simulink library "BaselineVehicleController_cl"  (R2020a)
settings: Solver=VariableStepAuto  StartTime=0.0  StopTime=10.0  RelTol=1e-3
undefined symbols (not defined in the file): best_gear, Clutch, dem_wheel_speed, dem_wheel_torque, Gear, ICE, MTC, Neg_RPM, Neg_T_eng_Nm, t_acc, tau_acc, TRAN, VEH
libraries: BaselineVelocityController_UL x1, Traffic_2_UL x1
settings Model: Creator=John Jr  LastModifiedBy=John Jr

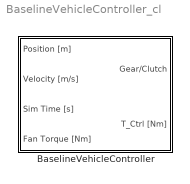
== system BaselineVehicleController_cl ==
  BaselineVehicleController : Subsystem

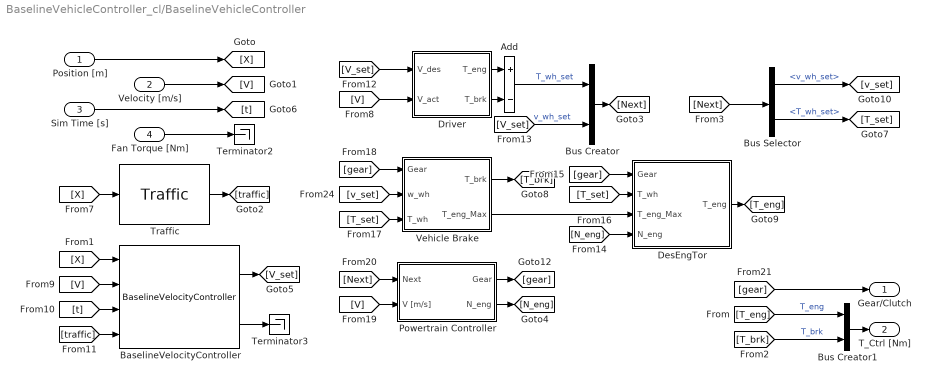
== system BaselineVehicleController_cl/BaselineVehicleController ==
  Position [m] : Inport
  Velocity [m/s] : Inport  Port=2
  Sim Time [s] : Inport  Port=3
  Fan Torque [Nm] : Inport  Port=4
  Add : Sum  Inputs=+-
  BaselineVelocityController : BaselineVelocityController_UL/BaselineVelocityController  SystemSampleTime=-1  Latency=0  AutoFrameSizeCalculation=off
  Bus Creator : BusCreator  Inputs=2
  Bus Creator1 : BusCreator  Inputs=2
  Bus Selector : BusSelector  OutputSignals=v_wh_set,T_wh_set
  DesEngTor : Subsystem
  Driver : Subsystem
  Powertrain Controller : Subsystem
  Terminator2 : Terminator
  Terminator3 : Terminator
  Traffic : Traffic_2_UL/Traffic  SystemSampleTime=-1  Latency=0  AutoFrameSizeCalculation=off
  Vehicle Brake : Subsystem
  Gear/Clutch : Outport  VectorParamsAs1DForOutWhenUnconnected=off
  T_Ctrl [Nm] : Outport  Port=2  VectorParamsAs1DForOutWhenUnconnected=off
  wires:
  Velocity [m/s]/1 -> [V]
  Position [m]/1 -> [X]
  Bus Selector/2 -> [T_set]  "<T_wh_set>"
  [Next] -> Bus Selector/1
  Bus Selector/1 -> [v_set]  "<v_wh_set>"
  Fan Torque [Nm]/1 -> Terminator2/1
  [gear] -> Gear/Clutch/1
  Bus Creator1/1 -> T_Ctrl [Nm]/1
  [X] -> Traffic/1
  Traffic/1 -> [traffic]
  Sim Time [s]/1 -> [t]
  [X] -> BaselineVelocityController/1
  [V] -> BaselineVelocityController/2
  [t] -> BaselineVelocityController/3
  [traffic] -> BaselineVelocityController/4
  Bus Creator/1 -> [Next]
  [V_set] -> Driver/1(V_des)
  [V_set] -> Bus Creator/2  "v_wh_set"
  Add/1 -> Bus Creator/1  "T_wh_set"
  Driver/2(T_brk) -> Add/2
  Driver/1(T_eng) -> Add/1
  [V] -> Driver/2(V_act)
  BaselineVelocityController/1 -> [V_set]
  BaselineVelocityController/2 -> Terminator3/1
  [gear] -> Vehicle Brake/1(Gear)
  [gear] -> DesEngTor/1(Gear)
  [v_set] -> Vehicle Brake/2(w_wh)
  Vehicle Brake/1(T_brk) -> [T_brk]
  [N_eng] -> DesEngTor/4(N_eng)
  [T_set] -> DesEngTor/2(T_wh)
  [T_set] -> Vehicle Brake/3(T_wh)
  Vehicle Brake/2(T_eng_Max) -> DesEngTor/3(T_eng_Max)
  DesEngTor/1(T_eng) -> [T_eng]
  [Next] -> Powertrain Controller/1(Next)
  Powertrain Controller/1(Gear) -> [gear]
  [V] -> Powertrain Controller/2(V [m/s])
  [T_eng] -> Bus Creator1/1  "T_eng"
  [T_brk] -> Bus Creator1/2  "T_brk"
  Powertrain Controller/2(N_eng) -> [N_eng]

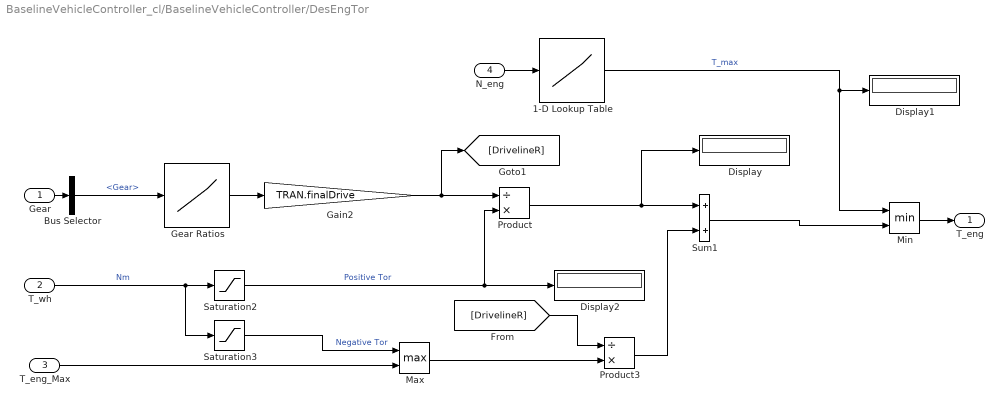
== system BaselineVehicleController_cl/BaselineVehicleController/DesEngTor ==
  Gear : Inport
  T_wh : Inport  Port=2
  T_eng_Max : Inport  Port=3
  N_eng : Inport  Port=4
  1-D Lookup Table : Lookup_n-D  NumberOfTableDimensions=1  BreakpointsForDimension1=MTC.espd  Table=MTC.T_max  InternalRulePriority=Speed  RndMeth=Simplest  InputSameDT=on
  Bus Selector : BusSelector  OutputSignals=Gear
  Display : Display
  Display1 : Display
  Display2 : Display
  Gain2 : Gain  Gain=TRAN.finalDrive
  Gear Ratios : Lookup_n-D  NumberOfTableDimensions=1  BreakpointsForDimension1=[1:TRAN.numGears]  Table=TRAN.gears  ExtrapMethod=Clip  UseLastTableValue=on  InternalRulePriority=Speed  RndMeth=Simplest  InputSameDT=on
  Max : MinMax  Function=max  Inputs=2
  Min : MinMax  Inputs=2
  Product : Product  Inputs=/*
  Product3 : Product  Inputs=/*
  Saturation2 : Saturate  UpperLimit=inf  LowerLimit=0
  Saturation3 : Saturate  UpperLimit=0  LowerLimit=-inf
  Sum1 : Sum
  T_eng : Outport  VectorParamsAs1DForOutWhenUnconnected=off
  wires:
  Gain2/1 -> [DrivelineR], Product/1
  Product/1 -> Display/1, Sum1/1
  T_wh/1 -> Saturation3/1, Saturation2/1  "Nm"
  Gear Ratios/1 -> Gain2/1
  Saturation2/1 -> Display2/1, Product/2  "Positive Tor"
  Saturation3/1 -> Max/1  "Negative Tor"
  Product3/1 -> Sum1/2
  T_eng_Max/1 -> Max/2
  Max/1 -> Product3/2
  [DrivelineR] -> Product3/1
  Gear/1 -> Bus Selector/1
  Bus Selector/1 -> Gear Ratios/1  "<Gear>"
  N_eng/1 -> 1-D Lookup Table/1
  Sum1/1 -> Min/2
  1-D Lookup Table/1 -> Display1/1, Min/1  "T_max"
  Min/1 -> T_eng/1

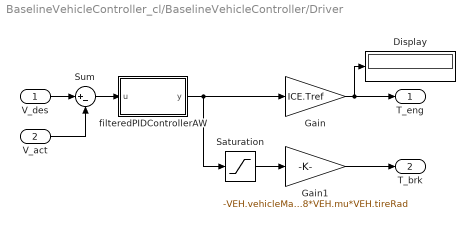
== system BaselineVehicleController_cl/BaselineVehicleController/Driver ==
  V_des : Inport
  V_act : Inport  Port=2
  Display : Display
  Gain : Gain  Gain=ICE.Tref
  Gain1 : Gain  Gain=-VEH.vehicleMass*9.8*VEH.mu*VEH.tireRad
  Saturation : Saturate  UpperLimit=0  LowerLimit=-1
  Sum : Sum  Inputs=|+-
  filteredPIDControllerAW : Subsystem  mask{kp=5, ki=1, kd=0, tau=.01, cmax=1, cmin=-1}
      mask prompts: kp "Proportional Gain, kp"; ki "Integral Gain, ki"; kd "Derivative Gain, kd"; tau "Time Constant, s"; cmax "Control Upper Limit"; cmin "Control Lower Limit"
  T_eng : Outport  VectorParamsAs1DForOutWhenUnconnected=off
  T_brk : Outport  Port=2  VectorParamsAs1DForOutWhenUnconnected=off
  wires:
  Sum/1 -> filteredPIDControllerAW/1(u)
  Saturation/1 -> Gain1/1
  V_des/1 -> Sum/1
  V_act/1 -> Sum/2
  Gain1/1 -> T_brk/1
  filteredPIDControllerAW/1(y) -> Saturation/1, Gain/1
  Gain/1 -> Display/1, T_eng/1

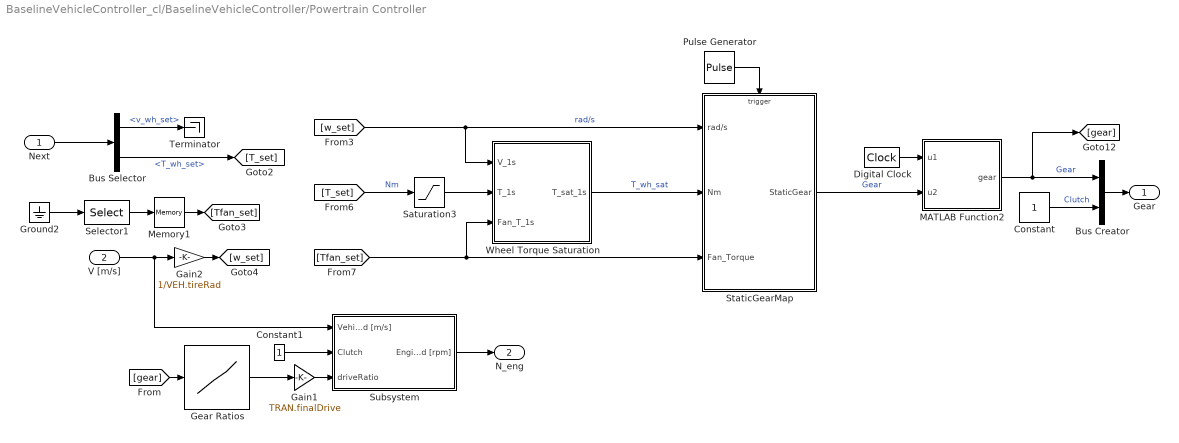
== system BaselineVehicleController_cl/BaselineVehicleController/Powertrain Controller ==
  Next : Inport
  V [m/s] : Inport  Port=2
  Bus Creator : BusCreator  Inputs=Gear,Clutch
  Bus Selector : BusSelector  OutputSignals=v_wh_set,T_wh_set
  Constant : Constant
  Constant1 : Constant
  Digital Clock : DigitalClock
  Gain1 : Gain  Gain=TRAN.finalDrive
  Gain2 : Gain  Gain=1/VEH.tireRad
  Gear Ratios : Lookup_n-D  NumberOfTableDimensions=1  BreakpointsForDimension1=[1:TRAN.numGears]  Table=TRAN.gears  ExtrapMethod=Clip  UseLastTableValue=on  InternalRulePriority=Speed  RndMeth=Simplest  InputSameDT=on
  Ground2 : Ground
  MATLAB Function2 : MATLAB Function  TreatAsAtomicUnit=on
  Memory1 : Memory  InheritSampleTime=on
  Pulse Generator : DiscretePulseGenerator  PulseType=Time based  Period=7
  Saturation3 : Saturate  UpperLimit=inf  LowerLimit=0
  Selector1 : Selector  InputPortWidth=1  IndexOptions=Index vector (dialog)  Indices=[1]  OutputSizes=1
  StaticGearMap : Subsystem
  Subsystem : Subsystem
  Terminator : Terminator
  Wheel Torque Saturation : Subsystem
  Gear : Outport  VectorParamsAs1DForOutWhenUnconnected=off
  N_eng : Outport  Port=2  VectorParamsAs1DForOutWhenUnconnected=off
  wires:
  MATLAB Function2/1(gear) -> [gear], Bus Creator/1  "Gear"
  Pulse Generator/1 -> StaticGearMap/Trigger
  [T_set] -> Saturation3/1  "Nm"
  Constant/1 -> Bus Creator/2  "Clutch"
  [w_set] -> Wheel Torque Saturation/1(V_1s), StaticGearMap/1(rad/s)  "rad/s"
  Bus Creator/1 -> Gear/1
  Next/1 -> Bus Selector/1
  Saturation3/1 -> Wheel Torque Saturation/2(T_1s)
  Wheel Torque Saturation/1(T_sat_1s) -> StaticGearMap/2(Nm)  "T_wh_sat"
  [Tfan_set] -> StaticGearMap/3(Fan_Torque), Wheel Torque Saturation/3(Fan_T_1s)
  Selector1/1 -> Memory1/1
  Bus Selector/2 -> [T_set]  "<T_wh_set>"
  Memory1/1 -> [Tfan_set]
  Digital Clock/1 -> MATLAB Function2/1(u1)
  StaticGearMap/1(StaticGear) -> MATLAB Function2/2(u2)  "Gear"
  Gain2/1 -> [w_set]
  Ground2/1 -> Selector1/1
  V [m/s]/1 -> Subsystem/1(Vehicle Speed [m/s]), Gain2/1
  Bus Selector/1 -> Terminator/1  "<v_wh_set>"
  Subsystem/1(Engine Speed [rpm]) -> N_eng/1
  Constant1/1 -> Subsystem/2(Clutch)
  Gear Ratios/1 -> Gain1/1
  Gain1/1 -> Subsystem/3(driveRatio)
  [gear] -> Gear Ratios/1

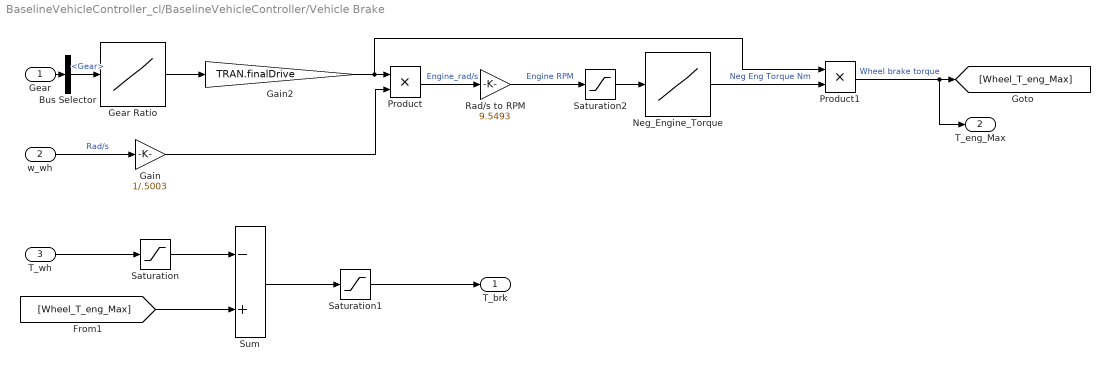
== system BaselineVehicleController_cl/BaselineVehicleController/Vehicle Brake ==
  Gear : Inport
  w_wh : Inport  Port=2
  T_wh : Inport  Port=3
  Bus Selector : BusSelector  OutputSignals=Gear
  Gain : Gain  Gain=1/.5003
  Gain2 : Gain  Gain=TRAN.finalDrive
  Gear Ratio : Lookup_n-D  NumberOfTableDimensions=1  BreakpointsForDimension1=[1 2 3 4 5 6 7 8 9 10 11 12]  BreakpointsForDimension2=[1:3]  Table=[11.73 9.21 7.09 5.57 4.34 3.41 2.69 2.12 1.63 1.28 1 0.7850]  InternalRulePriority=Speed  RndMeth=Simplest  InputSameDT=on
  Neg_Engine_Torque : Lookup_n-D  NumberOfTableDimensions=1  BreakpointsForDimension1=Neg_RPM  BreakpointsForDimension2=[1:3]  Table=Neg_T_eng_Nm  InternalRulePriority=Speed  RndMeth=Simplest  InputSameDT=on
  Product : Product
  Product1 : Product
  Rad/s to RPM : Gain  Gain=9.5493
  Saturation : Saturate  UpperLimit=0  LowerLimit=-inf
  Saturation1 : Saturate  UpperLimit=inf  LowerLimit=0
  Saturation2 : Saturate  UpperLimit=2100  LowerLimit=0
  Sum : Sum  Inputs=-+
  T_brk : Outport  VectorParamsAs1DForOutWhenUnconnected=off
  T_eng_Max : Outport  Port=2  VectorParamsAs1DForOutWhenUnconnected=off
  wires:
  Rad/s to RPM/1 -> Saturation2/1  "Engine RPM"
  Neg_Engine_Torque/1 -> Product1/2  "Neg Eng Torque Nm"
  Gear Ratio/1 -> Gain2/1
  Gain2/1 -> Product1/1, Product/1
  w_wh/1 -> Gain/1  "Rad/s"
  Product/1 -> Rad/s to RPM/1  "Engine_rad/s"
  Product1/1 -> T_eng_Max/1, [Wheel_T_eng_Max]  "Wheel brake torque"
  T_wh/1 -> Saturation/1
  [Wheel_T_eng_Max] -> Sum/2
  Saturation/1 -> Sum/1
  Sum/1 -> Saturation1/1
  Saturation1/1 -> T_brk/1
  Saturation2/1 -> Neg_Engine_Torque/1
  Bus Selector/1 -> Gear Ratio/1  "<Gear>"
  Gear/1 -> Bus Selector/1
  Gain/1 -> Product/2

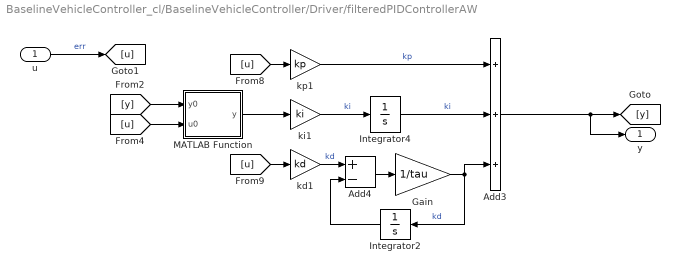
== system BaselineVehicleController_cl/BaselineVehicleController/Driver/filteredPIDControllerAW ==
  u : Inport  PortDimensions=1
  Add3 : Sum  Inputs=+++
  Add4 : Sum  Inputs=+-
  Gain : Gain  Gain=1/tau
  Integrator2 : Integrator
  Integrator4 : Integrator
  MATLAB Function : MATLAB Function  TreatAsAtomicUnit=on  mask{cMax=cmax, cMin=cmin}
      mask prompts: cMax "Max control value:"; cMin "Min control value:"
  kd1 : Gain  Gain=kd
  ki1 : Gain  Gain=ki
  kp1 : Gain  Gain=kp
  y : Outport  PortDimensions=1  VectorParamsAs1DForOutWhenUnconnected=off
  wires:
  [u] -> MATLAB Function/2(u0)
  [y] -> MATLAB Function/1(y0)
  u/1 -> [u]  "err"
  kd1/1 -> Add4/1  "kd"
  Integrator2/1 -> Add4/2
  Integrator4/1 -> Add3/2  "ki"
  kp1/1 -> Add3/1  "kp"
  Add4/1 -> Gain/1
  [u] -> kp1/1
  ki1/1 -> Integrator4/1  "ki"
  Gain/1 -> Add3/3, Integrator2/1  "kd"
  [u] -> kd1/1
  MATLAB Function/1(y) -> ki1/1
  Add3/1 -> y/1, [y]

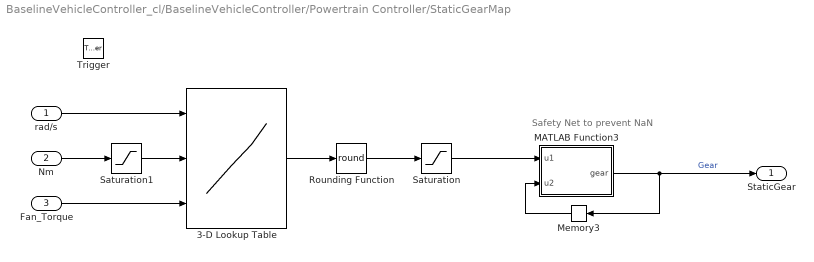
== system BaselineVehicleController_cl/BaselineVehicleController/Powertrain Controller/StaticGearMap ==
  note: Safety Net to prevent NaN
  rad/s : Inport
  Nm : Inport  Port=2
  Fan_Torque : Inport  Port=3
  Trigger : TriggerPort  VariantControl=Variant  PortDimensions=1
  3-D Lookup Table : Lookup_n-D  NumberOfTableDimensions=3  BreakpointsForDimension1=dem_wheel_speed  BreakpointsForDimension2=dem_wheel_torque  BreakpointsForDimension3=t_acc  Table=best_gear  InternalRulePriority=Speed  RndMeth=Simplest  InputSameDT=on
  MATLAB Function3 : MATLAB Function  TreatAsAtomicUnit=on
  Memory3 : Memory  InitialCondition=11  InheritSampleTime=on
  Rounding Function : Rounding  Operator=round
  Saturation : Saturate  UpperLimit=12  LowerLimit=1
  Saturation1 : Saturate  UpperLimit=inf  LowerLimit=0
  StaticGear : Outport  VectorParamsAs1DForOutWhenUnconnected=off
  wires:
  Fan_Torque/1 -> 3-D Lookup Table/3
  Rounding Function/1 -> Saturation/1
  Saturation1/1 -> 3-D Lookup Table/2
  Nm/1 -> Saturation1/1
  rad/s/1 -> 3-D Lookup Table/1
  3-D Lookup Table/1 -> Rounding Function/1
  Memory3/1 -> MATLAB Function3/2(u2)
  Saturation/1 -> MATLAB Function3/1(u1)
  MATLAB Function3/1(gear) -> StaticGear/1, Memory3/1  "Gear"

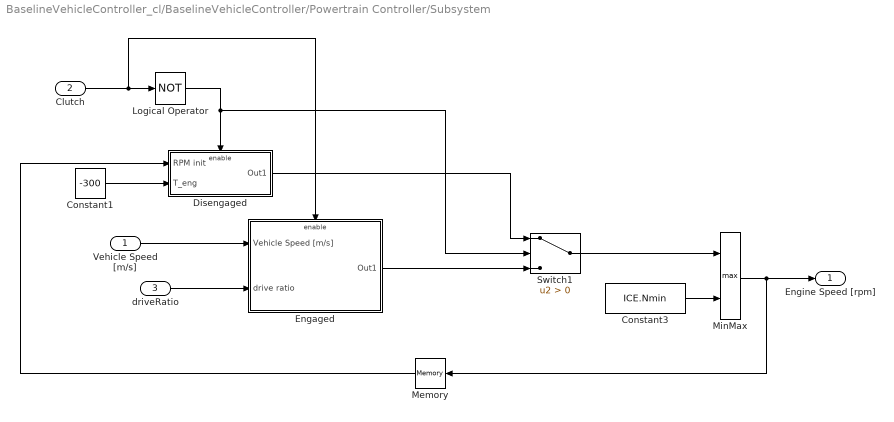
== system BaselineVehicleController_cl/BaselineVehicleController/Powertrain Controller/Subsystem ==
  Vehicle Speed [m/s] : Inport
  Clutch : Inport  Port=2
  driveRatio : Inport  Port=3
  Constant1 : Constant  Value=-300
  Constant3 : Constant  Value=ICE.Nmin
  Disengaged : Subsystem  TreatAsAtomicUnit=on
  Engaged : Subsystem  TreatAsAtomicUnit=on
  Logical Operator : Logic  Operator=NOT  AllPortsSameDT=off  OutDataTypeStr=boolean
  Memory : Memory  InitialCondition=ICE.Nmin
  MinMax : MinMax  Function=max  Inputs=2
  Switch1 : Switch  Criteria=u2 > Threshold
  Engine Speed [rpm] : Outport  VectorParamsAs1DForOutWhenUnconnected=off
  wires:
  Engaged/1(Out1) -> Switch1/3
  Memory/1 -> Disengaged/1(RPM init)
  Constant3/1 -> MinMax/2
  Switch1/1 -> MinMax/1
  MinMax/1 -> Engine Speed [rpm]/1, Memory/1
  driveRatio/1 -> Engaged/2(drive ratio)
  Vehicle Speed [m/s]/1 -> Engaged/1(Vehicle Speed [m/s])
  Logical Operator/1 -> Disengaged/Enable, Switch1/2
  Constant1/1 -> Disengaged/2(T_eng)
  Disengaged/1(Out1) -> Switch1/1
  Clutch/1 -> Logical Operator/1, Engaged/Enable

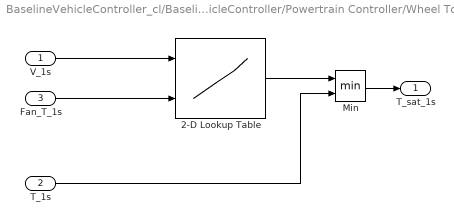
== system BaselineVehicleController_cl/BaselineVehicleController/Powertrain Controller/Wheel Torque Saturation ==
  V_1s : Inport
  T_1s : Inport  Port=2
  Fan_T_1s : Inport  Port=3
  2-D Lookup Table : Lookup_n-D  BreakpointsForDimension1=dem_wheel_speed  BreakpointsForDimension2=tau_acc  Table=WheelTorque_Max'  InternalRulePriority=Speed  RndMeth=Simplest  InputSameDT=on
  Min : MinMax  Inputs=2
  T_sat_1s : Outport  VectorParamsAs1DForOutWhenUnconnected=off
  wires:
  V_1s/1 -> 2-D Lookup Table/1
  Fan_T_1s/1 -> 2-D Lookup Table/2
  2-D Lookup Table/1 -> Min/1
  T_1s/1 -> Min/2
  Min/1 -> T_sat_1s/1

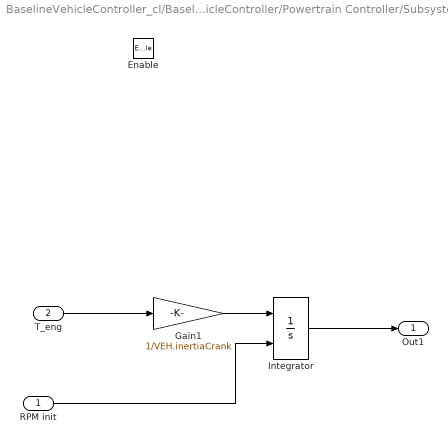
== system BaselineVehicleController_cl/BaselineVehicleController/Powertrain Controller/Subsystem/Disengaged ==
  RPM init : Inport
  T_eng : Inport  Port=2
  Enable : EnablePort  StatesWhenEnabling=reset
  Gain1 : Gain  Gain=1/VEH.inertiaCrank
  Integrator : Integrator  InitialConditionSource=external
  Out1 : Outport  InitialOutput=ICE.Nmin  VectorParamsAs1DForOutWhenUnconnected=off
  wires:
  RPM init/1 -> Integrator/2
  Gain1/1 -> Integrator/1
  T_eng/1 -> Gain1/1
  Integrator/1 -> Out1/1

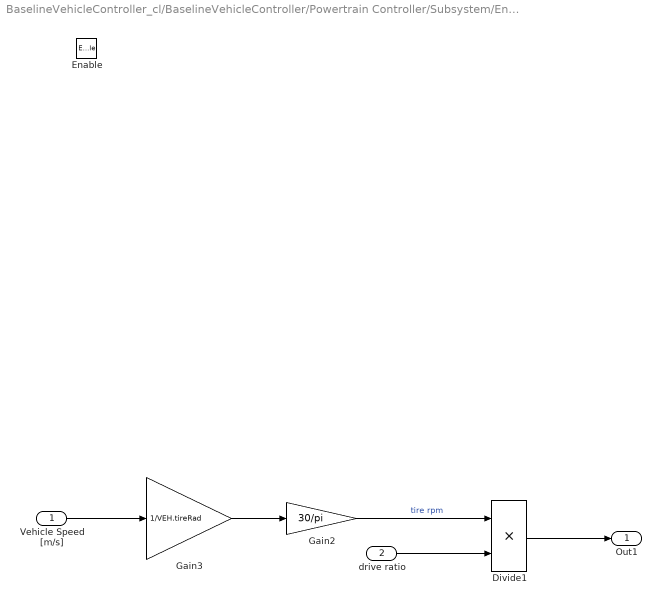
== system BaselineVehicleController_cl/BaselineVehicleController/Powertrain Controller/Subsystem/Engaged ==
  Vehicle Speed [m/s] : Inport
  drive ratio : Inport  Port=2
  Enable : EnablePort  StatesWhenEnabling=reset
  Divide1 : Product  Inputs=**
  Gain2 : Gain  Gain=30/pi
  Gain3 : Gain  Gain=1/VEH.tireRad
  Out1 : Outport  InitialOutput=ICE.Nmin  VectorParamsAs1DForOutWhenUnconnected=off
  wires:
  Divide1/1 -> Out1/1
  Vehicle Speed [m/s]/1 -> Gain3/1
  drive ratio/1 -> Divide1/2
  Gain3/1 -> Gain2/1
  Gain2/1 -> Divide1/1  "tire rpm"

== matlab function BaselineVehicleController_cl/BaselineVehicleController/Driver/filteredPIDControllerAW/MATLAB Function ==
  data: y0 input; u0 input; y output; cMax parameter; cMin parameter
function y = fcn(y0, u0, cMax, cMin)

if y0 > cMax
    y1 = cMax; 
elseif y0 < cMin
    y1 = cMin; 
else
    y1 = y0; 
end

sat = y0-y1; 
aw = exp(-1e5*sat^2); 
y = aw*u0;

== matlab function BaselineVehicleController_cl/BaselineVehicleController/Powertrain Controller/MATLAB Function2 ==
  data: u1 input; gear output; u2 input
function gear = fcn(u1, u2)
if u1 <= 7 
    gear=11;
else
    gear=u2;
end

== matlab function BaselineVehicleController_cl/BaselineVehicleController/Powertrain Controller/StaticGearMap/MATLAB Function3 ==
  data: u1 input; gear output; u2 input
function gear = fcn(u1, u2)
if isnan(u1)
    gear=u2;
else
    gear=u1;
end
